simulink model "xc"  (R2017b)
settings: Solver=VariableStepAuto  StartTime=0.0  StopTime=10.0  RelTol=1e-3
settings Model: Creator=jenkins  LastModifiedBy=jenkins
settings ConfigComp: CovEnable=on  RecordCoverage=on  CovModelRefEnable=on

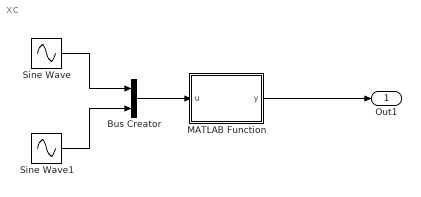
== system xc ==
  Bus Creator : BusCreator  Inputs=2
  MATLAB Function : MATLAB Function  TreatAsAtomicUnit=on
  Sine Wave : Sin  SampleTime=0
  Sine Wave1 : Sin  Amplitude=2  SampleTime=0
  Out1 : Outport
  wires:
  Sine Wave/1 -> Bus Creator/1
  Sine Wave1/1 -> Bus Creator/2
  Bus Creator/1 -> MATLAB Function/1(u)
  MATLAB Function/1(y) -> Out1/1

== matlab function xc/MATLAB Function ==
  data: u input; y output
function y = myXCorr(u)

y = xcorr(u(1), u(2), int32(1));
